simulink model "dynamics"  (R2023b)
settings: Solver=ode15s  StartTime=0.0  StopTime=8.6667  RelTol=1e-5
undefined symbols (not defined in the file or in its folder): f_fcn
settings Model: Creator=cosimodellasantina  LastModifiedBy=mrsub
settings SolverCC: AlgebraicLoopSolver=TrustRegion
settings DebuggingCC: UnconnectedInputMsg=warning  UnconnectedOutputMsg=warning  UnconnectedLineMsg=warning
settings ModelReferenceCC: EnableRefExpFcnMdlSchedulingChecks=on
settings SFSimCC: CustomCodeUndefinedFunction=UseInterfaceOnly
settings RTWCC: DLArmComputeVersion=19.05

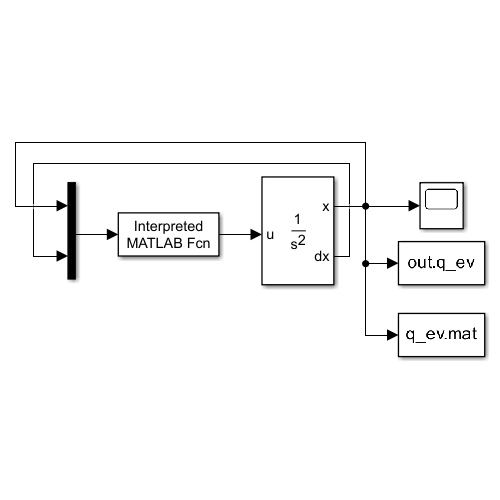
[thumbnail: Simulink's stored preview of the top-level diagram]
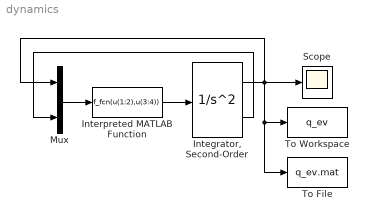
== system dynamics ==
  "Integrator, Second-Order" : SecondOrderIntegrator  ICX=x_0  ICDXDT=dx_0
  Interpreted MATLAB Function : MATLABFcn  MATLABFcn=f_fcn(u(1:2),u(3:4))
  Mux : Mux  Inputs=2
  Scope : Scope
  To File : ToFile  Filename=q_ev.mat  SaveFormat=Timeseries
  To Workspace : ToWorkspace  VariableName=q_ev  SaveFormat=Timeseries  SampleTime=-1
  wires:
  Mux/1 -> Interpreted MATLAB Function/1
  Interpreted MATLAB Function/1 -> "Integrator, Second-Order"/1
  "Integrator, Second-Order"/1 -> Mux/1, To File/1, To Workspace/1, Scope/1
  "Integrator, Second-Order"/2 -> Mux/2
